simulink model "Expriment_All2"  (R2014a)
settings: Solver=FixedStepDiscrete  SolverMode=SingleTasking  StartTime=0.0  StopTime=inf  FixedStep=0.01  RelTol=1e-3
PostLoadFcn:
  | h_RPStest = RPStest;
model workspace (MAT data in the model file):
  gtest = 0
undefined symbols (not defined in the file or in its folder): avert, avert_freq_factor, avert_gaze_dirs_chance, avert_gaze_duration_factor, avert_head_frequency_factor, avert_head_speed, BML, BML1, BML2, bmlsL, bmlsM, bodyBusyFlag, clock, emotion_amount_factor, faceBusyFlag, fileID, GAZE_WIN, gazing, mut_freq_factor, mutual_gaze_duration_factor, P, pose_cat_chance, pose_chanc_factor, pose_chance_factor, pose_frequency_factor, pose_lean, pose_lean_flag, pose_speed, pose_twitch, pr, serial, STATE_BEFORE, STATE_GO, STATE_OVER, STATE_READY, Stateflow
libraries: simulink x24, instrumentlib x6, lib_affectiveChar_behavior x2, realtime_pacer_lib x2, lib_affectiveChar_input x1
(part 6 of 7)

== stateflow chart Expriment_All2/CharacterControl/personalSpace_Controller ==
  state stateInit
    entry: gameState=14;
    TOO_CLOSE=1;TOO_FAR=2;NEUTRAL=0;
    farBuffer=0;closeBuffer=0;neutralBuffer=0;position=1;
    n=encStr2Arr(' ');bmlsM=[n n n n n];newBmlsM=[n n n n n];
    bmlsL=[n n n n n];newBmlsL=[n n n n n];
  note: Problem:
      | Sometimes locomotion BML is sent (visible in the vhmsgYarpRelais) but it is not running. Also smartbody shows duplicate msg id error. It seems that when too many BMLs are sent to smartbody some of them have same IDs.
  state wait
  note: if avert not 1
  state gazeSurprized
    entry: [P,BMLM]=walkInvadingTable(5) ;
    closeBuffer=closeBuffer+1;
    newBmlsM=insertQueue(bmlsM,BMLM);
    bmlsM=newBmlsM;
  state doIt3Times
    entry: position=2;
    closeBuffer=0;
  note: User is too close!
  state headNeuralGazeCamera
    entry: [P,BMLM]=walkInvadingTable(4) ;
    newBmlsM=insertQueue(bmlsM,BMLM);
    bmlsM=newBmlsM;
  state stateWalkBack
    entry:  [P,BMLM]=walkInvadingTable(2);
    newBmlsM=insertQueue(bmlsM,BMLM);  bmlsM=newBmlsM;
    closeBuffer=closeBuffer+1;
  state browUp
    entry: [P,BMLM]=walkInvadingTable(8) ;
    neutralBuffer=neutralBuffer+1;
    newBmlsM=insertQueue(bmlsM,BMLM);
    bmlsM=newBmlsM;
  state doIt3Times1
    entry: position=1;
    neutralBuffer=0;
  note: EXE ORDER IMPORTANT
  state checkUserCoord
  note: correct: [zChange==1]{position=0;}
  state idle
    entry: [P,BMLM]=walkInvadingTable(1);
    newBmlsM=insertQueue(bmlsM,BMLM);
    bmlsM=newBmlsM;
    neutralBuffer=neutralBuffer+1;
  note: User is in the middle!
  state wait2
  state leanFW
    entry: [P,BMLM]=walkInvadingTable(6) ;
    farBuffer=farBuffer+1;
    newBmlsM=insertQueue(bmlsM,BMLM);
    bmlsM=newBmlsM;
  state doIt3Times2
    entry: position=3;
    farBuffer=0;
  note: Problem:
      | We dont know where smatbody is standing (z pos). If smartbody does not run the locomotion BML sent for any reason (too many BMLs), we want to send locomodation BML again after a while to make sure the personal space is correct. On the other hand, we dont want the module to keep sending move bmls.
  state walkFW
    entry:  [P,BMLM]=walkInvadingTable(3) ;
    newBmlsM=insertQueue(bmlsM,BMLM);  bmlsM=newBmlsM;
    farBuffer=farBuffer+1;
  note: User is too far!
  state leanNeutral
    entry:  [P,BMLM]=walkInvadingTable(7) ;
    newBmlsM=insertQueue(bmlsM,BMLM); bmlsM=newBmlsM;
  (default) -> stateInit
  stateInit -> (junction 2)
  wait -> (junction 2)
  (junction 2) -> headNeuralGazeCamera [order 1] : [avert==1]
  (junction 2) -> checkUserCoord [order 2]
  idle -> wait [order 2] : after(5,secs)
  walkFW -> wait [order 2] : after(5,secs)
  stateWalkBack -> wait [order 2] : after(5,secs)
  doIt3Times1 -> wait : after(5,secs)
  doIt3Times2 -> wait : after(5,secs)
  doIt3Times -> wait : after(5,secs)
  checkUserCoord -> (junction 89) [order 3] : [[distance==TOO_CLOSE]&[position~=2]]
  (junction 89) -> gazeSurprized [order 2] : [closeBuffer<2]
  (junction 89) -> stateWalkBack [order 1] : [closeBuffer>=2]
  stateWalkBack -> doIt3Times [order 1] : [closeBuffer==5]
  gazeSurprized -> checkUserCoord
  headNeuralGazeCamera -> checkUserCoord
  checkUserCoord -> (junction 92) [order 2] : [[distance==NEUTRAL]&[position~=1]]
  (junction 92) -> browUp [order 1] : [neutralBuffer<2]
  wait2 -> checkUserCoord [order 1] : [zChange==1]{position=0;}
  idle -> doIt3Times1 [order 1] : [neutralBuffer==5]
  browUp -> checkUserCoord
  (junction 92) -> idle [order 2] : [neutralBuffer>=2]
  wait2 -> checkUserCoord [order 2] : [zChange~=1]
  checkUserCoord -> wait2 [order 4] : after(20,secs)
  checkUserCoord -> (junction 87) [order 1] : [[distance==TOO_FAR]&[position~=3]]
  leanFW -> checkUserCoord
  (junction 87) -> leanFW [order 2] : [farBuffer<2]
  walkFW -> doIt3Times2 [order 1] : [farBuffer==5]
  (junction 87) -> leanNeutral [order 1] : [farBuffer>=2]
  leanNeutral -> walkFW : after(2,secs)
  data: bmls function_input double size=[1000,5]; myBML function_input double size=[1000,1]; newBmls function_output double size=[1000,5]; p function_output double size=1; bmlID function_input double size=1; poseBML function_output double size=[1000,1]; bmls function_input double size=[1000,5]; myBML function_input double size=[1000,1]; newBmls function_output double size=[1000,5]; gameState output double size=1; STATE_READY data_store_memory size=1; STATE_OVER data_store_memory size=1; distance input double size=1; STATE_BEFORE data_store_memory size=1; BML1 data_store_memory size=[256,1]; P data_store_memory; pr data_store_memory; fileID data_store_memory; neutralBuffer local; closeBuffer local; NEUTRAL local; TOO_FAR local; TOO_CLOSE local; farBuffer local; zChange input; position local; avert data_store_memory; newBmlsM local double size=[1000,5]; bmlsM data_store_memory; BMLM local double size=[1000,1]; BMLL local double size=[1000,1]; newBmlsL local double size=[1000,5]; bmlsL data_store_memory; n local
  events: secs input RISING_EDGE_EVENT
  function newBmls =insertQueueLow(bmls,myBML):
    | function newBmls =insertQueueLow(bmls,myBML)
    |     full=1;
    |     t=encStr2Arr(' ');
    |     newBmls=[t t t t t];
    |     for i = 1:5
    |         if (isequal(bmls(:,i),t))
    |             %add to end of the queue where its empty
    |             bmls(:,i)=myBML;
    |             full=0;
    |             break
    |         end
    |     end
    |     if(full~=0)
    |             %if queue full, shift all elements to left which removes the first one, then add to end
    |             bmls(:,1)= bmls(:,2);
    |             bmls(:,2)= bmls(:,3);
    |             bmls(:,3)= bmls(:,4);
    |             bmls(:,5)=myBML;
    |     end
    |     newBmls=bmls;
  function [p,poseBML]=walkInvadingTable(bmlID):
    | function [p,poseBML]=walkInvadingTable(bmlID)
    | 
    | aVarTruthTableCondition_1 = false;
    | aVarTruthTableCondition_2 = false;
    | aVarTruthTableCondition_3 = false;
    | aVarTruthTableCondition_4 = false;
    | aVarTruthTableCondition_5 = false;
    | aVarTruthTableCondition_6 = false;
    | aVarTruthTableCondition_7 = false;
    | aVarTruthTableCondition_8 = false;
    | 
    | 
    | % n
    | 
    | aVarTruthTableCondition_1 = logical(bmlID==1);
    | 
    | % b
    | 
    | aVarTruthTableCondition_2 = logical(bmlID==2);
    | 
    | % f
    | 
    | aVarTruthTableCondition_3 = logical(bmlID==3);
    | 
    | % HN
    | 
    | aVarTruthTableCondition_4 = logical(bmlID==4);
    | 
    | % surprizeGaze
    | 
    | aVarTruthTableCondition_5 = logical(bmlID==5);
    | 
    | % leanFw
    | 
    | aVarTruthTableCondition_6 = logical(bmlID==6);
    | 
    | % leanNeutral
    | 
    | aVarTruthTableCondition_7 = logical(bmlID==7);
    | 
    | % browUp
    | 
    | aVarTruthTableCondition_8 = logical(bmlID==8);
    | 
    | if (aVarTruthTableCondition_1)
    |     aFcnTruthTableAction_1();
    | elseif (aVarTruthTableCondition_2)
    |     aFcnTruthTableAction_2();
    | elseif (aVarTruthTableCondition_3)
    |     aFcnTruthTableAction_3();
    | elseif (aVarTruthTableCondition_4)
    |     aFcnTruthTableAction_4();
    | elseif (aVarTruthTableCondition_5)
    |     aFcnTruthTableAction_5();
    | elseif (aVarTruthTableCondition_6)
    |     aFcnTruthTableAction_6();
    | elseif (aVarTruthTableCondition_7)
    |     aFcnTruthTableAction_7();
    | elseif (aVarTruthTableCondition_8)
    |     aFcnTruthTableAction_8();
    | else % Default
    |     aFcnTruthTableAction_1();
    | end
    | 
    | function aFcnTruthTableAction_1()
    | 
    | % Neutral
    | 
    | poseBML=encStr2Arr( '<?xml version="1.0" ?><act><bml><locomotion manner="walk" facing="gazeTarget"  sbm:accel="0.5" sbm:scootaccel="50" target="0 0"/></bml></act>');p=1;
    | 
    | function aFcnTruthTableAction_2()
    | 
    | % Back
    | 
    | poseBML=encStr2Arr( '<?xml version="1.0" ?><act><bml><locomotion manner="walk"  sbm:accel="0.5" sbm:scootaccel="50" facing="gazeTarget" target="0 -0.6"/></bml></act>');p=1;
    | 
    | function aFcnTruthTableAction_3()
    | 
    | % Forward
    | 
    | poseBML=encStr2Arr( '<?xml version="1.0" ?><act><bml><locomotion manner="walk" facing="gazeTarget"  sbm:accel="0.5" sbm:scootaccel="50" target="0 0.6"/></bml></act>');p=1;
    | 
    | function aFcnTruthTableAction_4()
    | 
    | % NeutralHead
    | 
    | poseBML=encStr2Arr('<?xml version="1.0" ?><act><bml><gaze target="gazeTarget" sbm:joint-range="EYES NECK" sbm:time-hint="1.5"/></bml></act>');p=1;
    | 
    | function aFcnTruthTableAction_5()
    | 
    | % surprisedGaze
    | 
    | poseBML=encStr2Arr('<?xml version="1.0" ?><act><bml><face type="FACS" start="0" end="5" side="BOTH" au="5" relax="3" amount="0.5"/><face type="FACS" start="0" end="5" side="BOTH" au="2" relax="3" amount="0.5"/></bml></act>');p=1;
    | 
    | function aFcnTruthTableAction_6()
    | 
    | % leanFW
    | 
    | poseBML=encStr2Arr('<?xml version="1.0" ?><act><bml><gaze angle="5" direction="DOWN" sbm:joint-range="HEAD BACK" sbm:time-hint="2" target="gazeTarget"/></bml></act>');p=1;
    | 
    | function aFcnTruthTableAction_7()
    | 
    | % leanNeutral
    | 
    | poseBML=encStr2Arr('<?xml version="1.0" ?><act><bml><gaze sbm:time-hint="2" target="gazeTarget"/></bml></act>');p=1;
    | 
    | function aFcnTruthTableAction_8()
    | 
    | % browUp
    | 
    | poseBML=encStr2Arr('<?xml version="1.0" ?><act><bml><face au="2" end="5" ready="1" relax="4" side="BOTH" start="0" stroke="3" type="facs"/></bml></act>');p=1;
  function newBmls =insertQueue(bmls,myBML):
    | function newBmls =insertQueue(bmls,myBML)
    |     full=1;
    |     t=encStr2Arr(' ');
    |     newBmls=[t t t t t];
    |     for i = 1:5
    |         if (isequal(bmls(:,i),t))
    |             %add to end of the queue where its empty
    |             bmls(:,i)=myBML;
    |             full=0;
    |             break
    |         end
    |     end
    |     if(full~=0)
    |             %if queue full, shift all elements to left which removes the first one, then add to end
    |             bmls(:,1)= bmls(:,2);
    |             bmls(:,2)= bmls(:,3);
    |             bmls(:,3)= bmls(:,4);
    |             bmls(:,5)=myBML;
    |     end
    |     newBmls=bmls;

== stateflow chart Expriment_All2/CharacterControl/attention_Controller ==
  state setBodyFlag [parallel]
    settings: executionOrder=1
    state wait
      entry: timer=20;
    state init
      entry: bodyBusyFlag=0;timer=1;
    state flagOne
      entry:  bodyBusyFlag=1;
    state check
    state flagZero
      entry: bodyBusyFlag=0;
    (default) -> init
    init -> check
    flagOne -> wait [order 1] : [body_isAttending==1]
    wait -> flagOne
    check -> flagOne : [body_isAttending==1]
    flagZero -> check
    flagOne -> flagZero [order 2] : after(timer,secs)
  state setFaceFlag [parallel]
    settings: executionOrder=2
    state wait2
      entry: timer2=10;
    state init2
      entry: faceBusyFlag=0;timer2=1;
    state flagOne2
      entry:  faceBusyFlag=1;
    state check2
    state flagZero2
      entry: faceBusyFlag=0;
    (default) -> init2
    init2 -> check2
    flagOne2 -> wait2 [order 1] : [face_isAttending==1]
    wait2 -> flagOne2
    check2 -> flagOne2 : [face_isAttending==1]
    flagZero2 -> check2
    flagOne2 -> flagZero2 [order 2] : after(timer2,secs)
  data: bodyBusyFlag data_store_memory size=1; body_isAttending input; timer local; face_isAttending input; faceBusyFlag data_store_memory size=1; timer2 local
  events: secs input RISING_EDGE_EVENT

== stateflow chart Expriment_All2/CharacterControl/emotion_Behavior_Factors ==
  state init
    entry: mutual_gaze_duration_factor=1;avert_gaze_duration_factor=1;avert_head_frequency_factor=20;avert_head_speed=1;avert_gaze_dirs_chance=0;,avert_freq_factor=1;mut_freq_factor=1;
    pose_frequency_factor=40;pose_chanc_factor=1;pose_cat_chance=50;pose_lean=18;pose_speed=1;pose_lean_flag=0; pose_space=0; blink_flag=0; blinkperiod_min=5;blinkperiod_max=9;
  state wait
  state setBehavior
    entry:
    [mutual_gaze_duration_factor, avert_gaze_duration_factor,avert_head_frequency_factor,avert_head_speed,avert_gaze_dirs_chance,avert_freq_factor,mut_freq_factor,blink_flag, blinkperiod_min,blinkperiod_max]=sharedFunc.setGazeFactors(inV,inA,personality,personalityFlag,vaFlag,gazeArray,personalityChange);
    [pose_twitch,pose_frequency_factor,pose_chanc_factor,pose_cat_chance,pose_lean,pose_speed,pose_lean_flag,pose_space]=sharedFunc.setPoseFactors(inV,inA,personality,personalityFlag,vaFlag,poseArray,personalityChange);
  state sharedFunc [group]
  (default) -> init
  init -> wait
  wait -> setBehavior [order 2] : [vChange==1]
  wait -> setBehavior [order 1] : [aChange==1]
  setBehavior -> wait
  data: inA input double size=1; inV input double size=1; personality input; gazeArray input; aChange input; personalityFlag input; vaFlag input; avert_head_frequency_factor data_store_memory; avert_gaze_duration_factor data_store_memory; mutual_gaze_duration_factor data_store_memory; avert_head_speed data_store_memory; avert_gaze_dirs_chance data_store_memory; poseArray input; pose_lean data_store_memory; pose_speed data_store_memory; pose_lean_flag data_store_memory; pose_cat_chance data_store_memory; pose_frequency_factor data_store_memory; pose_chanc_factor data_store_memory; personalityChange input; avert_freq_factor data_store_memory; mut_freq_factor data_store_memory; pose_twitch data_store_memory; vChange input; blinkperiod_min data_store_memory; blinkperiod_max data_store_memory; blink_flag data_store_memory; pose_space data_store_memory

== matlab function Expriment_All2/EmotionSubsystem/calculateValenceArousal/HEHN_A ==
  data: a2 output double size=1; a1 input double size=1
function a2 = fcn(a1)

aVarTruthTableCondition_1 = false;
aVarTruthTableCondition_2 = false;



aVarTruthTableCondition_1 = logical(a1>10);


aVarTruthTableCondition_2 = logical(a1<-10);

if (aVarTruthTableCondition_1)
    aFcnTruthTableAction_1();
elseif (aVarTruthTableCondition_2)
    aFcnTruthTableAction_2();
else % Default
    aFcnTruthTableAction_3();
end

function aFcnTruthTableAction_1()


a2=a1;

function aFcnTruthTableAction_2()


a2=a1;

function aFcnTruthTableAction_3()


a2=0;

== matlab function Expriment_All2/EmotionSubsystem/calculateValenceArousal/HELN_A ==
  data: a2 output double size=1; a1 input double size=1
function a2 = fcn(a1)

aVarTruthTableCondition_1 = false;
aVarTruthTableCondition_2 = false;



aVarTruthTableCondition_1 = logical(a1>10);


aVarTruthTableCondition_2 = logical(a1<-10);

if (aVarTruthTableCondition_1)
    aFcnTruthTableAction_1();
elseif (aVarTruthTableCondition_2)
    aFcnTruthTableAction_2();
else % Default
    aFcnTruthTableAction_3();
end

function aFcnTruthTableAction_1()


a2=a1;

function aFcnTruthTableAction_2()


a2=a1;

function aFcnTruthTableAction_3()


a2=0;

== matlab function Expriment_All2/EmotionSubsystem/arousalFlagFunction ==
  data: userInvade input; interactionState input; a_trig output; a_trigW output; vaFlag input; randa input
function [a_trig,a_trigW]= fcn(userInvade,interactionState,vaFlag,randa)
%#codegen
% 30/06/2015
    %Here set in which states of the interaction agent experienced 
    % more arousal(arousalFlag=1) and less arousal (arousalFlag=-1)
    %Note that you should define the states in your scenraio beforehand
    %we assume agent gets more aroused when in ready/go state and 
    %less aroused when in WAITE/HAND
    if(vaFlag==1)
        a_trigW=0; %weight by which arousal value is changed (sum of weight of all triggers)

        %randa 30% chance of random increase or decrease in arousal
        randTrigger=floor(randa);
        if(0<randTrigger)&&(randTrigger<30)
            a_trigW=a_trigW + 0.6;
        end
        if(30<randTrigger)&&(randTrigger<60)
            a_trigW=a_trigW - 0.6;
        end

        if(interactionState==1)%GO - highely aroused state
            a_trigW=a_trigW+0.5;
        end
        if(interactionState==7)%READY - high aroused state
            a_trigW=a_trigW+0.5;
        end
        if(interactionState==2)%HAND- highely aroused state
            a_trigW=a_trigW -0.5;
        end
        if(interactionState==6)%WAIT - low aroused state
            a_trigW=a_trigW-0.5;
        end
        %     elseif(interactionState==3)%OVER - low aroused state
    %         arousalTrig=-1;  
    %         end
        if(userInvade==1)
           a_trigW=a_trigW+0.25;
        end
    else
        a_trigW=0;
    end
    if(a_trigW>0)
        a_trig=1;
    elseif(a_trigW<0)
        a_trig=-1;
        a_trigW=abs(a_trigW);
    else
        a_trig=0;
    end

== matlab function Expriment_All2/randomArray/makleArray ==
  data: r1 input; y output double size=[1,40]; r2 input; r3 input; r4 input; r5 input; r6 input; r7 input; r8 input; r9 input; r10 input; r11 input; r12 input; r13 input; r14 input; r15 input; r16 input; r17 input; r18 input; r19 input; r20 input; r21 input; r22 input; r23 input; r24 input; r25 input; r26 input; r27 input; r28 input; r29 input; r30 input; r31 input; r32 input; r33 input; r34 input; r35 input; r36 input; r37 input; r38 input; r39 input; r40 input
function y = fcn(r1,r2,r3,r4,r5,r6,r7,r8,r9,r10,r11,r12,r13,r14,r15,r16, r17, r18, r19,r20,r21,r22,r23,r24,r25,r26,r27,r28,r29,r30,r31,r32,r33,r34,r35,r36,r37,r38,r39,r40)
%#codegen
y=[0,0,0,0,0,0,0,0,0,0,  0,0,0,0,0,0,0,0,0,0,  0,0,0,0,0,0,0,0,0,0,  0,0,0,0,0,0,0,0,0,0];
y(:,1) = floor(r1);
y(:,2) = floor(r2);
y(:,3) = floor(r3);
y(:,4) = floor(r4);
y(:,5) = floor(r5);
y(:,6) = floor(r6);
y(:,7) = floor(r7);
y(:,8) = floor(r8);
y(:,9) = floor(r9);
y(:,10) = floor(r10);
y(:,11) = floor(r11);
y(:,12) = floor(r12);
y(:,13) = floor(r13);
y(:,14) = floor(r14);
y(:,15) = floor(r15);
y(:,16) = floor(r16);
y(:,17) = floor(r17);
y(:,18) = floor(r18);
y(:,19) = floor(r19);
y(:,20) = floor(r20);
y(:,21) = floor(r21);
y(:,22) = floor(r22);
y(:,23) = floor(r23);
y(:,24) = floor(r24);
y(:,25) = floor(r25);
y(:,26) = floor(r26);
y(:,27) = floor(r27);
y(:,28) = floor(r28);
y(:,29) = floor(r29);
y(:,30) = floor(r30);
y(:,31) = floor(r31);
y(:,32) = floor(r32);
y(:,33) = floor(r33);
y(:,34) = floor(r34);
y(:,35) = floor(r35);
y(:,36) = floor(r36);
y(:,37) = floor(r37);
y(:,38) = floor(r37);
y(:,39) = floor(r39);
y(:,40) = floor(r40);

== stateflow chart Expriment_All2/CharacterControl/wave_Controller ==
  state init
    entry: STATE_OVER=3;
    STATE_BEFORE=4;
    gameState=14;
    rFlag=0;lFlag=0;bFlag=0;
    n=encStr2Arr(' ');bmlsM=[n n n n n];
    newBmlsM=[n n n n n];
  state waveRightHand
    entry: [P,BMLM]= wavePoseBradTable(1+animNum);
    rFlag=1;
    newBmlsM=insertQueue(bmlsM,BMLM);
    bmlsM=newBmlsM;
  state gazeCamera
    entry: [P,BMLM]= wavePoseBradTable(8);
    avert=0;
    newBmlsM=insertQueue(bmlsM,BMLM);
    bmlsM=newBmlsM;
  state wave
    entry: animNum =setPersonalityParams(personality);
  state waveLeftHand
    entry:
    [P,BMLM]= wavePoseBradTable(animNum);
    lFlag=1;
    newBmlsM=insertQueue(bmlsM,BMLM);
    bmlsM=newBmlsM;
  state gazeCamera1
    entry: [P,BMLM]= wavePoseBradTable(8);
    avert=0;
    newBmlsM=insertQueue(bmlsM,BMLM);
    bmlsM=newBmlsM;
  note: if introvert 50% chance of introvertWave(poseN=7)
  note: else(extrovert)
  state gazeCamera2
    entry: [P,BMLM]= wavePoseBradTable(8);
    avert=0;
    newBmlsM=insertQueue(bmlsM,BMLM);
    bmlsM=newBmlsM;
  state waveBothHands
    entry: [P,BMLM]= wavePoseBradTable(3+animNum);
    bFlag=1;
    newBmlsM=insertQueue(bmlsM,BMLM);
    bmlsM=newBmlsM;
  note: Problem with procedural behaviors (you can not give duration and they stay in that pose untill new bml comes so they dont return to idle)
      | we want the agent to gaze at user for the period of waving.If new idle gaze BML comes, agent averts gaze or head before wave finished. Gaze is procedural (gazes at the point till new gaze bml is recieved so it does not automatically return to idle pose) so we can not give duration of gaze in the BML. The only way to avoid avert during wave is to make sure thre is no idle gaze bmls during the wave; which makes sense considering the gaze does not avert(idle) when you are attending something.
      | prioritizing does not solve this because avertGaze comes right after gazeCamera and wave. We also can not delay after high priorities because sometime several high priorities should happen right after eachother.
  waveBothHands -> wave : after(5,secs)
  waveRightHand -> wave : after(5,secs)
  waveLeftHand -> wave : after(5,secs)
  (default) -> init
  init -> wave
  (junction 55) -> waveRightHand [order 2]
  gazeCamera -> waveRightHand : after(2,secs)
  wave -> (junction 55) [order 4] : [[handUp==1]&[rFlag==0]]{ lFlag=0;bFlag=0;}
  (junction 55) -> gazeCamera [order 1] : [avert==1]
  wave -> wave [order 1] : after(10,secs){ rFlag=0;lFlag=0;bFlag=0;}
  wave -> (junction 59) [order 3] : [[handUp==3]&[bFlag==0]]{ rFlag=0;lFlag=0;}
  wave -> (junction 58) [order 2] : [[handUp==2]&[lFlag==0]]{ rFlag=0;bFlag=0;}
  (junction 82) -> waveLeftHand [order 1] : [randP==1]{animNum=7;}
  (junction 58) -> (junction 79) [order 2]
  (junction 79) -> (junction 82) [order 1] : [[personality==2]|[personality==4]]{randP=randArray(:,12)}
  (junction 58) -> gazeCamera1 [order 1] : [avert==1]
  gazeCamera1 -> (junction 79) : after(2,secs)
  (junction 79) -> waveLeftHand [order 2] : {animNum=2+animNum;}
  (junction 82) -> waveLeftHand [order 2] : [randP==2]{animNum=2+animNum;}
  (junction 59) -> waveBothHands [order 2]
  (junction 59) -> gazeCamera2 [order 1] : [avert==1]
  gazeCamera2 -> waveBothHands : after(2,secs)
  data: pr function_output double size=1; bmlID function_input double; poseBML function_output double size=[1000,1]; num function_output double size=1; p function_input double size=1; bmls function_input double size=[1000,5]; mBML function_input double size=[1000,1]; newBmls function_output double size=[1000,5]; fileID data_store_memory; handUp input; gameState output double size=1; BML data_store_memory; P data_store_memory; STATE_OVER data_store_memory; STATE_BEFORE data_store_memory; rFlag local; lFlag local; bFlag local; BML2 data_store_memory; avert data_store_memory; BMLM local double size=[1000,1]; newBmlsM local double size=[1000,5]; bmlsM data_store_memory; n local; personality input double size=1; randP local; animNum local; randArray input double size=[1,40]; personalityChange input boolean size=1
  events: secs input RISING_EDGE_EVENT
  function [pr,poseBML]=wavePoseBradTable(bmlID):
    | function [pr,poseBML]=wavePoseBradTable(bmlID)
    | 
    | aVarTruthTableCondition_1 = false;
    | aVarTruthTableCondition_2 = false;
    | aVarTruthTableCondition_3 = false;
    | aVarTruthTableCondition_4 = false;
    | aVarTruthTableCondition_5 = false;
    | aVarTruthTableCondition_6 = false;
    | aVarTruthTableCondition_7 = false;
    | aVarTruthTableCondition_8 = false;
    | aVarTruthTableCondition_9 = false;
    | aVarTruthTableCondition_10 = false;
    | 
    | 
    | 
    | aVarTruthTableCondition_1 = logical(bmlID==1);
    | 
    | 
    | aVarTruthTableCondition_2 = logical(bmlID==2);
    | 
    | 
    | aVarTruthTableCondition_3 = logical(bmlID==3);
    | 
    | 
    | aVarTruthTableCondition_4 = logical(bmlID==4);
    | 
    | 
    | aVarTruthTableCondition_5 = logical(bmlID==5);
    | 
    | 
    | aVarTruthTableCondition_6 = logical(bmlID==6);
    | 
    | 
    | aVarTruthTableCondition_7 = logical(bmlID==7);
    | 
    | 
    | aVarTruthTableCondition_8 = logical(bmlID==8);
    | 
    | 
    | aVarTruthTableCondition_9 = logical(bmlID==9);
    | 
    | 
    | aVarTruthTableCondition_10 = logical(bmlID==10);
    | 
    | if (aVarTruthTableCondition_1)
    |     aFcnTruthTableAction_1();
    | elseif (aVarTruthTableCondition_2)
    |     aFcnTruthTableAction_2();
    | elseif (aVarTruthTableCondition_3)
    |     aFcnTruthTableAction_3();
    | elseif (aVarTruthTableCondition_4)
    |     aFcnTruthTableAction_4();
    | elseif (aVarTruthTableCondition_5)
    |     aFcnTruthTableAction_5();
    | elseif (aVarTruthTableCondition_6)
    |     aFcnTruthTableAction_6();
    | elseif (aVarTruthTableCondition_7)
    |     aFcnTruthTableAction_7();
    | elseif (aVarTruthTableCondition_8)
    |     aFcnTruthTableAction_8();
    | elseif (aVarTruthTableCondition_9)
    |     aFcnTruthTableAction_9();
    | elseif (aVarTruthTableCondition_10)
    |     aFcnTruthTableAction_10();
    | else % Default
    |     aFcnTruthTableAction_1();
    | end
    | 
    | function aFcnTruthTableAction_1()
    | 
    | % waveLeftF
    | 
    | poseBML=encStr2Arr('<?xml version="1.0" ?><act><bml><animation name="../data/ChrBrad/test_wave_left.skm" speed="2"/></bml></act>'); pr=2;
    | 
    | function aFcnTruthTableAction_2()
    | 
    | % waveRightF
    | 
    | poseBML=encStr2Arr('<?xml version="1.0" ?><act><bml><animation name="../data/ChrBrad/test_wave_right.skm" speed="2"/></bml></act>'); pr=2;
    | 
    | function aFcnTruthTableAction_3()
    | 
    | % waveBothF
    | 
    | poseBML=encStr2Arr('<?xml version="1.0" ?><act><bml><animation name="ChrBrad@Idle01_BeatHighBt01" speed="2"/></bml></act>'); pr=2;
    | 
    | function aFcnTruthTableAction_4()
    | 
    | % waveLeftSlow
    | 
    | poseBML=encStr2Arr('<?xml version="1.0" ?><act><bml><animation name="../data/ChrBrad/test_wave_left.skm" speed="0.5"/></bml></act>'); pr=2;
    | 
    | function aFcnTruthTableAction_5()
    | 
    | % WaveRightSlow
    | 
    | poseBML=encStr2Arr('<?xml version="1.0" ?><act><bml><animation name="../data/ChrBrad/test_wave_right.skm" speed="0.5"/></bml></act>'); pr=2;
    | 
    | function aFcnTruthTableAction_6()
    | 
    | % WaveBothSlow
    | 
    | poseBML=encStr2Arr('<?xml version="1.0" ?><act><bml><animation name="ChrBrad@Idle01_BeatHighBt01" speed="0.5"/></bml></act>'); pr=2;
    | 
    | function aFcnTruthTableAction_7()
    | 
    | % WaveLIntrovert
    | 
    | poseBML=encStr2Arr('<?xml version="1.0" ?><act><bml><animation name="../data/ChrBrad/test_introvert_wave.skm" speed="1"/></bml></act>'); pr=2;
    | 
    | function aFcnTruthTableAction_8()
    | 
    | % gazeCamera
    | 
    | poseBML=encStr2Arr('<?xml version="1.0" ?><act><bml><gaze target="gazeTarget" sbm:joint-range="EYES NECK" sbm:time-hint="1.5"/></bml></act>');pr=2;
    | 
    | function aFcnTruthTableAction_9()
    | 
    | % waveLeft
    | 
    | poseBML=encStr2Arr('<?xml version="1.0" ?><act><bml><animation name="ChrBrad@Idle01_BeatHighRt01"/></bml></act>');pr=2;
    | 
    | function aFcnTruthTableAction_10()
    | 
    | % waveRight
    | 
    | poseBML=encStr2Arr('<?xml version="1.0" ?><act><bml><animation name="ChrBrad@Idle01_BeatHighRt01"/></bml></act>');pr=2;
  function num =setPersonalityParams(p):
    | function num =setPersonalityParams(p)
    |  num=0;
    |  if(p==1) %HE
    |     num=0;
    |  elseif(p==2)%LE
    |     num=3;
    |  elseif(p==3)%HE
    |     num=0;
    |  else%LE
    |     num=3;
    |  end
  function newBmls =insertQueue(bmls,mBML):
    | function newBmls =insertQueue(bmls,mBML)
    |     full=1;
    |     t=encStr2Arr(' ');
    |     newBmls=[t t t t t];
    |     for i = 1:5
    |         if (isequal(bmls(:,i),t))
    |             %add to end of the queue where its empty
    |             bmls(:,i)=mBML;
    |             full=0;
    |             break
    |         end
    |     end
    |     if(full~=0)
    |             %if queue full, shift all elements to left which removes the first one, then add to end
    |                         disp('before add when full');disp(bmls);
    |             bmls(:,1)= bmls(:,2);
    |             bmls(:,2)= bmls(:,3);
    |             bmls(:,3)= bmls(:,4);
    |             bmls(:,5)=mBML;
    |             
    |     end
    |     newBmls=bmls;

== matlab function Expriment_All2/facialExpr/facialExprGen/matlabFuncIf/reset ==
  data: L input; u1 input; y output
function y = fcn(L,u1)
if(u1<=L)
    y= u1;
else
    y =1;
end

== matlab function Expriment_All2/facialExpr/facialExprGen/matlabFuncIf/displayBMLs ==
  data: e input; l input; i input double size=1 [1..]; bml input
function fcn(e,l,i,bml)
%#codegen
fprintf('%s','e:');fprintf('%f',e);
fprintf('%s','  ,L:');fprintf('%f',l);
fprintf('%s','  ,i:');fprintf('%f',i);
disp(decArr2Str(bml));

== matlab function Expriment_All2/facialExpr/facialExprGen/matlabFuncIf/plusOne ==
  data: y output; i input double size=1
function y  = iCheck(i)
%#codegen
    y=i+1;

== matlab function Expriment_All2/facialExpr/facialExprGen/matlabFuncIf/makeBmls ==
  data: i input double size=1 [1..]; arrAU input; eAmount input; arrBML output
function arrBML = fcn(i,arrAU,eAmount)
    %#codegen
    coder.extrinsic('sprintf');
    coder.extrinsic('strcat');
    
    %Maryam, 14-10-2015
    %'strcat' dimension 2  maximum size is 453,it was not possible to concat and send all bmls 
    %for one emotion together(used simulink for loop )    
    
    AU=arrAU(i);eA=eAmount(i);   
    c1 = countDigits(AU);c2 = countDigits(eA);

    str1 = sprintf('<?xml version=\"1.0\" ?><act><bml>');
    
    if(max(ceil(log10(abs(AU))),1)==1) %if AU is one-digit
        temp = sprintf('<face type=\"FACS\" side=\"BOTH\" au=\"%1d\"  start=\"0\" ready=\"1\" stroke=\"2\"  relax=\"300\" end=\"400\" amount=\"%0.1f\"/>',AU,eA); 
        temp2=strcat(str1,temp);
        str1=temp2;
    else      
        temp = sprintf('<face type=\"FACS\" side=\"BOTH\" au=\"%2d\" start=\"0\" ready=\"1\" stroke=\"2\"  relax=\"300\" end=\"400\" amount=\"%0.1f\"/>',AU,eA);
        temp2=strcat(str1,temp);
        str1=temp2;
    end

    str2 = sprintf('</bml></act>');
    %n=length(arrAU);
    %mystr=blanks(arrAU(n));
    mystr=blanks(142+c1+c2);
    mystr = strcat (str1,str2);    
    arrBML = encStr2Arr(mystr);

== stateflow chart Expriment_All2/GazeFollowSubsystem/resetGazeTarget/createGazePawn ==
  state sendSBM(In2) [function]
  state stateCreatePawn
    entry:
    sendSBM(encStr2Arr('scene.getPawn(\"gazeTarget\").setPosition(SrVec(0,1.6,10))'));
  (default) -> stateCreatePawn
  data: In2 function_input double size=[1000 1]

== matlab function Expriment_All2/chack_E_Change1/checkNeutral ==
  data: notNeutral output double size=1; e input
function notNeutral = fcn(e)
%#codegen

if(e~=6)
    notNeutral=1;
else
    notNeutral=0;
end

== matlab function Expriment_All2/setPersonality ==
  data: extrovert input; personality output; neurotic input
function personality = fcn(extrovert,neurotic)
%#codegen
% 1 HEHN 2 LEHN 3 HELN 4 LELN
if(extrovert==1)
    if(neurotic==1)
        personality = 1;% 1 HEHN
    else 
        personality = 3;%HELN
    end
else
    if(neurotic==1)
        personality = 2;%LEHN
    else
        personality = 4;%LELN
    end
end

== matlab function Expriment_All2/EmotionSubsystem/calculateValenceArousal/HEHN_VA_Emo ==
  data: V input; e output double size=1; A input double
function e = fcn(V, A)

aVarTruthTableCondition_1 = false;
aVarTruthTableCondition_2 = false;
aVarTruthTableCondition_3 = false;
aVarTruthTableCondition_4 = false;
aVarTruthTableCondition_5 = false;
aVarTruthTableCondition_6 = false;
aVarTruthTableCondition_7 = false;
aVarTruthTableCondition_8 = false;


% 7-happy  2,1

aVarTruthTableCondition_1 = logical(V>10 && A<40 && A>10);

% 8-ex  1,2 AND 2,2

aVarTruthTableCondition_2 = logical(V>0 && A>40);

% 4-fear  -1,2 AND -2,2

aVarTruthTableCondition_3 = logical(V<0 && A>40);

% 3-frust  -2,1

aVarTruthTableCondition_4 = logical(V<-10 && A<40 && A>10);

% 6-pleased  2,-1

aVarTruthTableCondition_5 = logical(V>10 && A<-10 && A>-40);

% 5-calm  1,-2 AND 2,-2

aVarTruthTableCondition_6 = logical(V>0 && A<-40);

% 1-bored  -1,-2 AND -2,-2

aVarTruthTableCondition_7 = logical(V<0 && A<-40);

% 2-sad  -2,-1

aVarTruthTableCondition_8 = logical(V<-10 && A<-10 && A>-40);

if (aVarTruthTableCondition_1)
    aFcnTruthTableAction_1();
elseif (aVarTruthTableCondition_2)
    aFcnTruthTableAction_2();
elseif (aVarTruthTableCondition_3)
    aFcnTruthTableAction_3();
elseif (aVarTruthTableCondition_4)
    aFcnTruthTableAction_4();
elseif (aVarTruthTableCondition_5)
    aFcnTruthTableAction_5();
elseif (aVarTruthTableCondition_6)
    aFcnTruthTableAction_6();
elseif (aVarTruthTableCondition_7)
    aFcnTruthTableAction_7();
elseif (aVarTruthTableCondition_8)
    aFcnTruthTableAction_8();
else % Default
    aFcnTruthTableAction_5();
end

function aFcnTruthTableAction_1()

% happy

e=7;

function aFcnTruthTableAction_2()

% excited

e=8;

function aFcnTruthTableAction_3()

% fear

e=4;

function aFcnTruthTableAction_4()

% frustration

e=3;

function aFcnTruthTableAction_5()

% pleased

e=6;

function aFcnTruthTableAction_6()

% contempt

e=5;

function aFcnTruthTableAction_7()

% bored

e=1;

function aFcnTruthTableAction_8()

% sad

e=2;

== matlab function Expriment_All2/gazeInputArray/makeGazeArray ==
  data: r1 input; y output double size=[1,6]; r2 input; r3 input; r4 input; r5 input; r6 input
function y = fcn(r1,r2,r3,r4,r5,r6)
%#codegen
y=[0,0,0,0,0,0];
y(:,1) = floor(r1);
y(:,2) = floor(r2);
y(:,3) = floor(r3);
y(:,4) = floor(r4);
y(:,5) = floor(r5);
y(:,6) = floor(r6);

== matlab function Expriment_All2/EmotionSubsystem/calculateValenceArousal/LEHN_VA_Emo ==
  data: V input; e output double size=1; A input double
function e = fcn(V, A)

aVarTruthTableCondition_1 = false;
aVarTruthTableCondition_2 = false;
aVarTruthTableCondition_3 = false;
aVarTruthTableCondition_4 = false;
aVarTruthTableCondition_5 = false;
aVarTruthTableCondition_6 = false;
aVarTruthTableCondition_7 = false;
aVarTruthTableCondition_8 = false;


% 7-happy  2,1

aVarTruthTableCondition_1 = logical(V>20 && A<40 && A>20);

% 8-ex  1,2 AND 2,2

aVarTruthTableCondition_2 = logical(V>0 && A>40);

% 4-fear  -1,2 AND -2,2

aVarTruthTableCondition_3 = logical(V<0 && A>40);

% 3-frust  -2,1

aVarTruthTableCondition_4 = logical(V<-20 && A<40 && A>20);

% 6-idle  2,-1

aVarTruthTableCondition_5 = logical(V>20 && A<-20 && A>-40);

% 5-calm  1,-2 AND 2,-2

aVarTruthTableCondition_6 = logical(V>0 && A<-40);

% 1-bored  -1,-2 AND -2,-2

aVarTruthTableCondition_7 = logical(V<0 && A<-40);

% 2-sad  -2,-1

aVarTruthTableCondition_8 = logical(V<-20 && A<-20 && A>-40);

if (aVarTruthTableCondition_1)
    aFcnTruthTableAction_1();
elseif (aVarTruthTableCondition_2)
    aFcnTruthTableAction_2();
elseif (aVarTruthTableCondition_3)
    aFcnTruthTableAction_3();
elseif (aVarTruthTableCondition_4)
    aFcnTruthTableAction_4();
elseif (aVarTruthTableCondition_5)
    aFcnTruthTableAction_5();
elseif (aVarTruthTableCondition_6)
    aFcnTruthTableAction_6();
elseif (aVarTruthTableCondition_7)
    aFcnTruthTableAction_7();
elseif (aVarTruthTableCondition_8)
    aFcnTruthTableAction_8();
else % Default
    aFcnTruthTableAction_5();
end

function aFcnTruthTableAction_1()

% happy

e=7;

function aFcnTruthTableAction_2()

% excited

e=8;

function aFcnTruthTableAction_3()

% fear

e=4;

function aFcnTruthTableAction_4()

% frustration

e=3;

function aFcnTruthTableAction_5()

% idle

e=6;

function aFcnTruthTableAction_6()

% contempt

e=5;

function aFcnTruthTableAction_7()

% bored

e=1;

function aFcnTruthTableAction_8()

% sad

e=2;

== matlab function Expriment_All2/EmotionSubsystem/calculateValenceArousal/LEHN_A ==
  data: a2 output double size=1; a1 input double size=1
function a2 = fcn(a1)

aVarTruthTableCondition_1 = false;
aVarTruthTableCondition_2 = false;



aVarTruthTableCondition_1 = logical(a1>25);


aVarTruthTableCondition_2 = logical(a1<-25);

if (aVarTruthTableCondition_1)
    aFcnTruthTableAction_1();
elseif (aVarTruthTableCondition_2)
    aFcnTruthTableAction_2();
else % Default
    aFcnTruthTableAction_3();
end

function aFcnTruthTableAction_1()


a2=a1;

function aFcnTruthTableAction_2()


a2=a1;

function aFcnTruthTableAction_3()


a2=0;

== matlab function Expriment_All2/poseInputArray/makePoseArray ==
  data: r1 input; y output double size=[1,6]; r2 input; r3 input; r4 input; r5 input; r6 input
function y = fcn(r1,r2,r3,r4,r5,r6)
%#codegen
y=[0,0,0,0,0,0];
y(:,1) = floor(r1);
y(:,2) = floor(r2);
y(:,3) = floor(r3);
y(:,4) = floor(r4);
y(:,5) = floor(r5);
y(:,6) = floor(r6);

== matlab function Expriment_All2/EmotionSubsystem/calculateValenceArousal/HEHN plot ==
  data: v input; a input
function fcn(v,a)
%coder.extrinsic to bypass code generation
coder.extrinsic('fscanf')
coder.extrinsic('get_param');
% coder.extrinsic('importdata');

currentTime=get_param('Expriment_FacialExpr','SimulationTime');%use name of simulink proj

A = [v;a;currentTime];
fileID = fopen('HEHN_VA_table.txt','a');
fprintf(fileID,'%0.1f,%0.1f,%0.1f\r\n',A);
fclose(fileID);

% matrix = importdata('HEHN_VA_table.txt',','); 
% tri = delaunay(matrix(:,1),matrix(:,2));
% trisurf(tri,matrix(:,1),matrix(:,2),matrix(:,3))
% shading interp
% colorbar

%-----------------------------------------
% fileID = fopen('HEHN_VA_table.txt','r');
% formatSpec = '%1f\r %1f\r %1f\r\n';
% sizeA = [3 Inf];
% A = fscanf(fileID,formatSpec,sizeA)
% % A = A'
% fclose(fileID);

% x = zeros(100,2);y = zeros(100,2);
% filename = 'HEHN_VA_table.txt';
% delimiterIn = ' ';
% headerlinesIn = 1;
% A = importdata(filename,delimiterIn,headerlinesIn);

% fileID=fopen('HEHN_VA_table4.txt');
% s=textscan(fileID,'%d %d %d','headerlines',23);
% fclose(fileID);
% x=s{1}

== matlab function Expriment_All2/EmotionSubsystem/calculateValenceArousal/LEHN plot ==
  data: v input; a input
function fcn(v,a)
%coder.extrinsic to bypass code generation
coder.extrinsic('fscanf')
coder.extrinsic('get_param');
% coder.extrinsic('importdata');

currentTime=get_param('Expriment_FacialExpr','SimulationTime');%use name of simulink proj

A = [v;a;currentTime];

fileID = fopen('LEHN_VA_table.txt','a');
fprintf(fileID,'%0.1f,%0.1f,%0.1f\r\n',A);
fclose(fileID);

%use the following to draw the plot
%tmp_data = importdata('HEHN_VA_table.txt',','); 
%no need: x=tmp_data(:,1);y=tmp_data(:,2);z=tmp_data(:,3)
%matrix=tmp_data
%tri = delaunay(matrix(:,1),matrix(:,2));
%trisurf(tri,matrix(:,1),matrix(:,2),matrix(:,3))
%shading interp

%-----------------------------------------
% fileID = fopen('HEHN_VA_table.txt','r');
% formatSpec = '%1f\r %1f\r %1f\r\n';
% sizeA = [3 Inf];
% A = fscanf(fileID,formatSpec,sizeA)
% % A = A'
% fclose(fileID);

% x = zeros(100,2);y = zeros(100,2);
% filename = 'HEHN_VA_table.txt';
% delimiterIn = ' ';
% headerlinesIn = 1;
% A = importdata(filename,delimiterIn,headerlinesIn);

% fileID=fopen('HEHN_VA_table4.txt');
% s=textscan(fileID,'%d %d %d','headerlines',23);
% fclose(fileID);
% x=s{1}

== matlab function Expriment_All2/EmotionSubsystem/calculateValenceArousal/LELN plot ==
  data: v input; a input
function fcn(v,a)
%coder.extrinsic to bypass code generation
coder.extrinsic('fscanf')
coder.extrinsic('get_param');
% coder.extrinsic('importdata');

currentTime=get_param('Expriment_FacialExpr','SimulationTime');%use name of simulink proj

A = [v;a;currentTime];

fileID = fopen('LELN_VA_table.txt','a');
fprintf(fileID,'%0.1f,%0.1f,%0.1f\r\n',A);
fclose(fileID);

%use the following to draw the plot
%matrix = importdata('HEHN_VA_table.txt',','); 
%tri = delaunay(matrix(:,1),matrix(:,2));
%trisurf(tri,matrix(:,1),matrix(:,2),matrix(:,3))
%shading interp
%colorbar
%-----------------------------------------
% fileID = fopen('HEHN_VA_table.txt','r');
% formatSpec = '%1f\r %1f\r %1f\r\n';
% sizeA = [3 Inf];
% A = fscanf(fileID,formatSpec,sizeA)
% % A = A'
% fclose(fileID);

% x = zeros(100,2);y = zeros(100,2);
% filename = 'HEHN_VA_table.txt';
% delimiterIn = ' ';
% headerlinesIn = 1;
% A = importdata(filename,delimiterIn,headerlinesIn);

% fileID=fopen('HEHN_VA_table4.txt');
% s=textscan(fileID,'%d %d %d','headerlines',23);
% fclose(fileID);
% x=s{1}

== matlab function Expriment_All2/EmotionSubsystem/calculateValenceArousal/HELN_V ==
  data: v2 output double size=1; v1 input double size=1
function v2 = fcn(v1)

aVarTruthTableCondition_1 = false;
aVarTruthTableCondition_2 = false;



aVarTruthTableCondition_1 = logical(v1>10);


aVarTruthTableCondition_2 = logical(v1<-10);

if (aVarTruthTableCondition_1)
    aFcnTruthTableAction_1();
elseif (aVarTruthTableCondition_2)
    aFcnTruthTableAction_2();
else % Default
    aFcnTruthTableAction_3();
end

function aFcnTruthTableAction_1()


v2=v1;

function aFcnTruthTableAction_2()


v2=v1;

function aFcnTruthTableAction_3()


v2=0;

== matlab function Expriment_All2/EmotionSubsystem/calculateValenceArousal/LELN_V ==
  data: v2 output double size=1; v1 input double size=1
function v2 = fcn(v1)

aVarTruthTableCondition_1 = false;
aVarTruthTableCondition_2 = false;



aVarTruthTableCondition_1 = logical(v1>25);


aVarTruthTableCondition_2 = logical(v1<-25);

if (aVarTruthTableCondition_1)
    aFcnTruthTableAction_1();
elseif (aVarTruthTableCondition_2)
    aFcnTruthTableAction_2();
else % Default
    aFcnTruthTableAction_3();
end

function aFcnTruthTableAction_1()


v2=v1;

function aFcnTruthTableAction_2()


v2=v1;

function aFcnTruthTableAction_3()


v2=0;
